simulink model "SecRwRtStBkReclnTrgtPosSelc"  (R2018b)
settings: Solver=FixedStepDiscrete  StartTime=0.0  StopTime=10.0  FixedStep=0.01  RelTol=1e-3
undefined symbols (not defined in the file or in its folder): KeSMSw4SAcsMd23SecRwRtStBkReclnUpwdDnwdPos_Val, KeSMSw4SAcsMd23SecRwRtStBkReclnUpwdDnwdPosMax_Val, KeSMSw4SAcsMd23SecRwRtStBkReclnUpwdDnwdPosMin_Val, KeSMSw4SAcsMd24SecRwRtStBkReclnUpwdDnwdPos1_Val, KeSMSw4SAcsMd24SecRwRtStBkReclnUpwdDnwdPos2_Val, KeSMSw4SAcsMd24SecRwRtStBkReclnUpwdDnwdPosMax1_Val, KeSMSw4SAcsMd24SecRwRtStBkReclnUpwdDnwdPosMax2_Val, KeSMSw4SAcsMd24SecRwRtStBkReclnUpwdDnwdPosMin1_Val, KeSMSw4SAcsMd24SecRwRtStBkReclnUpwdDnwdPosMin2_Val, KeSMSw4SAcsMd25SecRwRtStBkReclnUpwdDnwdPos_Val, KeSMSw4SAcsMd25SecRwRtStBkReclnUpwdDnwdPosMax_Val, KeSMSw4SAcsMd25SecRwRtStBkReclnUpwdDnwdPosMin_Val, KeSMSw4SAcsMd26SecRwRtStBkReclnUpwdDnwdPos_Val, KeSMSw4SAcsMd26SecRwRtStBkReclnUpwdDnwdPosMax_Val, KeSMSw4SAcsMd26SecRwRtStBkReclnUpwdDnwdPosMin_Val, KeSMSw4sLyingMDSecRwRtStBkReclnUpwdDnwdPos_Val, KeSMSw4sLyingMDSecRwRtStBkReclnUpwdDnwdPosMax_Val, KeSMSw4sLyingMDSecRwRtStBkReclnUpwdDnwdPosMin_Val, KeSMSw4sRecoveryMDSecRwRtStBkReclnUpwdDnwdPos_Val, KeSMSw4sRecoveryMDSecRwRtStBkReclnUpwdDnwdPosMax_Val, KeSMSw4sRecoveryMDSecRwRtStBkReclnUpwdDnwdPosMin_Val, KeSMSw4sVIPMDSecRwRtStBkReclnUpwdDnwdPos_Val, KeSMSw4sVIPMDSecRwRtStBkReclnUpwdDnwdPosMax_Val, KeSMSw4sVIPMDSecRwRtStBkReclnUpwdDnwdPosMin_Val, KeSMSw6sAcsEntrySecRwRtStBkReclnUpwdDnwd1Pos_Val, KeSMSw6sAcsEntrySecRwRtStBkReclnUpwdDnwdPos1Max_Val, KeSMSw6sAcsEntrySecRwRtStBkReclnUpwdDnwdPos1Min_Val, KeSMSw6sAcsEntrySecRwRtStBkReclnUpwdDnwdPos_Val, KeSMSw6sAcsEntrySecRwRtStBkReclnUpwdDnwdPosMax_Val, KeSMSw6sAcsEntrySecRwRtStBkReclnUpwdDnwdPosMin_Val, KeSMSw6sAcsExtSecRwRtStBkReclnUpwdDnwdPos_Val, KeSMSw6sAcsExtSecRwRtStBkReclnUpwdDnwdPosMax_Val, KeSMSw6sAcsExtSecRwRtStBkReclnUpwdDnwdPosMin_Val, KeSMSw6sRecoveryMdSecRwRtStBkReclnUpwdDnwdPos_Val, KeSMSw6sRecoveryMdSecRwRtStBkReclnUpwdDnwdPosMax_Val, KeSMSw6sRecoveryMdSecRwRtStBkReclnUpwdDnwdPosMin_Val, KeSMSw6sVIPSecRwRtStBkReclnUpwdDnwdPos_Val, KeSMSw6sVIPSecRwRtStBkReclnUpwdDnwdPosMax_Val, KeSMSw6sVIPSecRwRtStBkReclnUpwdDnwdPosMin_Val, KeSMSwAcsEntrySecRwRtStBkReclnUpwdDnwdPos1_Val, KeSMSwAcsEntrySecRwRtStBkReclnUpwdDnwdPos1Max_Val, KeSMSwAcsEntrySecRwRtStBkReclnUpwdDnwdPos1Min_Val, KeSMSwAcsEntrySecRwRtStBkReclnUpwdDnwdPos_Val, KeSMSwAcsEntrySecRwRtStBkReclnUpwdDnwdPosMax_Val, KeSMSwAcsEntrySecRwRtStBkReclnUpwdDnwdPosMin_Val, KeSMSwAcsExtSecRwRtStBkReclnUpwdDnwdPos_Val, KeSMSwAcsExtSecRwRtStBkReclnUpwdDnwdPosMax_Val, KeSMSwAcsExtSecRwRtStBkReclnUpwdDnwdPosMin_Val, KeSMSwAcsMd32SecRwRtStBkReclnUpwdDnwdPos1_Val, KeSMSwAcsMd32SecRwRtStBkReclnUpwdDnwdPos1Max_Val, KeSMSwAcsMd32SecRwRtStBkReclnUpwdDnwdPos1Min_Val, KeSMSwAcsMd32SecRwRtStBkReclnUpwdDnwdPos_Val, KeSMSwAcsMd32SecRwRtStBkReclnUpwdDnwdPosMax_Val, KeSMSwAcsMd32SecRwRtStBkReclnUpwdDnwdPosMin_Val, KeSMSwAcsMd53SecRwRtStBkReclnUpwdDnwdPos1_Val, KeSMSwAcsMd53SecRwRtStBkReclnUpwdDnwdPos1Max_Val, KeSMSwAcsMd53SecRwRtStBkReclnUpwdDnwdPos1Min_Val, KeSMSwAcsMd53SecRwRtStBkReclnUpwdDnwdPos_Val, KeSMSwAcsMd53SecRwRtStBkReclnUpwdDnwdPosMax_Val, KeSMSwAcsMd53SecRwRtStBkReclnUpwdDnwdPosMin_Val ... (+12)
libraries: TrgtPosSelcLib x15, simulink x2
(part 2 of 2)

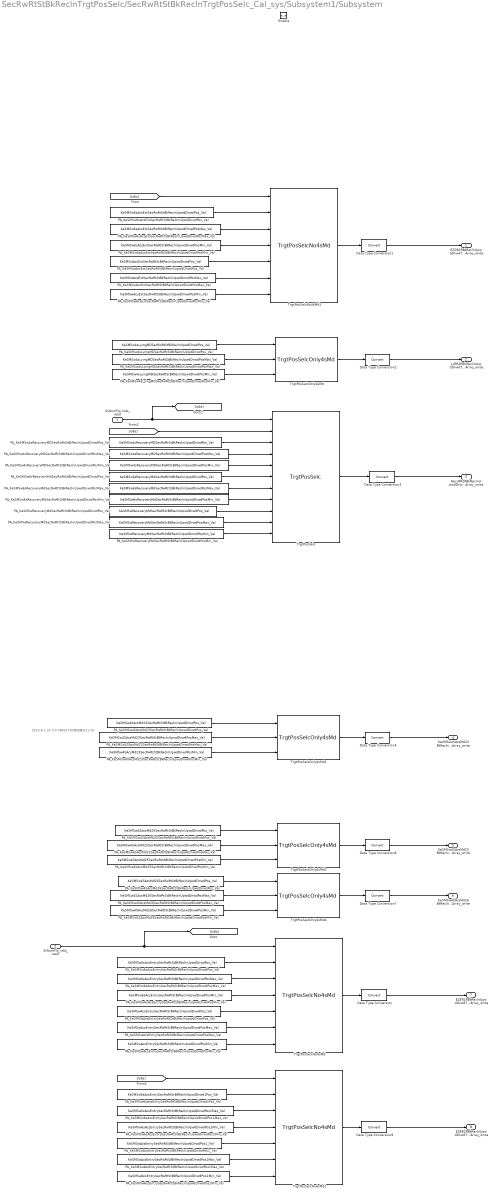
== system SecRwRtStBkReclnTrgtPosSelc/SecRwRtStBkReclnTrgtPosSelc_Cal_sys/Subsystem1/Subsystem ==
  note: 2023.8.1 V2.0.0 CR401790 增加模式21-26
  StNumFlg_Is4s_read : Inport
  StNumFlg_Is6s_read : Inport  Port=2
  Enable : EnablePort
  Data Type Conversion{,1..3,5..8} (8 alike) : DataTypeConversion
  PA_KeSMSw4SAcsMd23SecRwRtStBkReclnUpwdDnwdPosMax_Val : Constant  Value=KeSMSw4SAcsMd23SecRwRtStBkReclnUpwdDnwdPosMax_Val
  PA_KeSMSw4SAcsMd23SecRwRtStBkReclnUpwdDnwdPosMin_Val : Constant  Value=KeSMSw4SAcsMd23SecRwRtStBkReclnUpwdDnwdPosMin_Val
  PA_KeSMSw4SAcsMd23SecRwRtStBkReclnUpwdDnwdPos_Val : Constant  Value=KeSMSw4SAcsMd23SecRwRtStBkReclnUpwdDnwdPos_Val
  PA_KeSMSw4SAcsMd25SecRwRtStBkReclnUpwdDnwdPosMax_Val : Constant  Value=KeSMSw4SAcsMd25SecRwRtStBkReclnUpwdDnwdPosMax_Val
  PA_KeSMSw4SAcsMd25SecRwRtStBkReclnUpwdDnwdPosMin_Val : Constant  Value=KeSMSw4SAcsMd25SecRwRtStBkReclnUpwdDnwdPosMin_Val
  PA_KeSMSw4SAcsMd25SecRwRtStBkReclnUpwdDnwdPos_Val : Constant  Value=KeSMSw4SAcsMd25SecRwRtStBkReclnUpwdDnwdPos_Val
  PA_KeSMSw4SAcsMd26SecRwRtStBkReclnUpwdDnwdPosMax_Val : Constant  Value=KeSMSw4SAcsMd26SecRwRtStBkReclnUpwdDnwdPosMax_Val
  PA_KeSMSw4SAcsMd26SecRwRtStBkReclnUpwdDnwdPosMin_Val : Constant  Value=KeSMSw4SAcsMd26SecRwRtStBkReclnUpwdDnwdPosMin_Val
  PA_KeSMSw4SAcsMd26SecRwRtStBkReclnUpwdDnwdPos_Val : Constant  Value=KeSMSw4SAcsMd26SecRwRtStBkReclnUpwdDnwdPos_Val
  PA_KeSMSw4sLyingMDSecRwRtStBkReclnUpwdDnwdPosMax_Val : Constant  Value=KeSMSw4sLyingMDSecRwRtStBkReclnUpwdDnwdPosMax_Val
  PA_KeSMSw4sLyingMDSecRwRtStBkReclnUpwdDnwdPosMin_Val : Constant  Value=KeSMSw4sLyingMDSecRwRtStBkReclnUpwdDnwdPosMin_Val
  PA_KeSMSw4sLyingMDSecRwRtStBkReclnUpwdDnwdPos_Val : Constant  Value=KeSMSw4sLyingMDSecRwRtStBkReclnUpwdDnwdPos_Val
  PA_KeSMSw4sRecoveryMDSecRwRtStBkReclnUpwdDnwdPosMax_Val : Constant  Value=KeSMSw4sRecoveryMDSecRwRtStBkReclnUpwdDnwdPosMax_Val
  PA_KeSMSw4sRecoveryMDSecRwRtStBkReclnUpwdDnwdPosMin_Val : Constant  Value=KeSMSw4sRecoveryMDSecRwRtStBkReclnUpwdDnwdPosMin_Val
  PA_KeSMSw4sRecoveryMDSecRwRtStBkReclnUpwdDnwdPos_Val : Constant  Value=KeSMSw4sRecoveryMDSecRwRtStBkReclnUpwdDnwdPos_Val
  PA_KeSMSw6sAcsEntrySecRwRtStBkReclnUpwdDnwd1Pos_Val : Constant  Value=KeSMSw6sAcsEntrySecRwRtStBkReclnUpwdDnwd1Pos_Val
  PA_KeSMSw6sAcsEntrySecRwRtStBkReclnUpwdDnwdPos1Max_Val : Constant  Value=KeSMSw6sAcsEntrySecRwRtStBkReclnUpwdDnwdPos1Max_Val
  PA_KeSMSw6sAcsEntrySecRwRtStBkReclnUpwdDnwdPos1Min_Val : Constant  Value=KeSMSw6sAcsEntrySecRwRtStBkReclnUpwdDnwdPos1Min_Val
  PA_KeSMSw6sAcsEntrySecRwRtStBkReclnUpwdDnwdPosMax_Val : Constant  Value=KeSMSw6sAcsEntrySecRwRtStBkReclnUpwdDnwdPosMax_Val
  PA_KeSMSw6sAcsEntrySecRwRtStBkReclnUpwdDnwdPosMin_Val : Constant  Value=KeSMSw6sAcsEntrySecRwRtStBkReclnUpwdDnwdPosMin_Val
  PA_KeSMSw6sAcsEntrySecRwRtStBkReclnUpwdDnwdPos_Val : Constant  Value=KeSMSw6sAcsEntrySecRwRtStBkReclnUpwdDnwdPos_Val
  PA_KeSMSw6sAcsExtSecRwRtStBkReclnUpwdDnwdPosMax_Val : Constant  Value=KeSMSw6sAcsExtSecRwRtStBkReclnUpwdDnwdPosMax_Val
  PA_KeSMSw6sAcsExtSecRwRtStBkReclnUpwdDnwdPosMin_Val : Constant  Value=KeSMSw6sAcsExtSecRwRtStBkReclnUpwdDnwdPosMin_Val
  PA_KeSMSw6sAcsExtSecRwRtStBkReclnUpwdDnwdPos_Val : Constant  Value=KeSMSw6sAcsExtSecRwRtStBkReclnUpwdDnwdPos_Val
  PA_KeSMSw6sRecoveryMdSecRwRtStBkReclnUpwdDnwdPosMax_Val : Constant  Value=KeSMSw6sRecoveryMdSecRwRtStBkReclnUpwdDnwdPosMax_Val
  PA_KeSMSw6sRecoveryMdSecRwRtStBkReclnUpwdDnwdPosMin_Val : Constant  Value=KeSMSw6sRecoveryMdSecRwRtStBkReclnUpwdDnwdPosMin_Val
  PA_KeSMSw6sRecoveryMdSecRwRtStBkReclnUpwdDnwdPos_Val : Constant  Value=KeSMSw6sRecoveryMdSecRwRtStBkReclnUpwdDnwdPos_Val
  PA_KeSMSwAcsEntrySecRwRtStBkReclnUpwdDnwdPos1Max_Val : Constant  Value=KeSMSwAcsEntrySecRwRtStBkReclnUpwdDnwdPos1Max_Val
  PA_KeSMSwAcsEntrySecRwRtStBkReclnUpwdDnwdPos1Min_Val : Constant  Value=KeSMSwAcsEntrySecRwRtStBkReclnUpwdDnwdPos1Min_Val
  PA_KeSMSwAcsEntrySecRwRtStBkReclnUpwdDnwdPos1_Val : Constant  Value=KeSMSwAcsEntrySecRwRtStBkReclnUpwdDnwdPos1_Val
  PA_KeSMSwAcsEntrySecRwRtStBkReclnUpwdDnwdPosMax_Val : Constant  Value=KeSMSwAcsEntrySecRwRtStBkReclnUpwdDnwdPosMax_Val
  PA_KeSMSwAcsEntrySecRwRtStBkReclnUpwdDnwdPosMin_Val : Constant  Value=KeSMSwAcsEntrySecRwRtStBkReclnUpwdDnwdPosMin_Val
  PA_KeSMSwAcsEntrySecRwRtStBkReclnUpwdDnwdPos_Val : Constant  Value=KeSMSwAcsEntrySecRwRtStBkReclnUpwdDnwdPos_Val
  PA_KeSMSwAcsExtSecRwRtStBkReclnUpwdDnwdPosMax_Val : Constant  Value=KeSMSwAcsExtSecRwRtStBkReclnUpwdDnwdPosMax_Val
  PA_KeSMSwAcsExtSecRwRtStBkReclnUpwdDnwdPosMin_Val : Constant  Value=KeSMSwAcsExtSecRwRtStBkReclnUpwdDnwdPosMin_Val
  PA_KeSMSwAcsExtSecRwRtStBkReclnUpwdDnwdPos_Val : Constant  Value=KeSMSwAcsExtSecRwRtStBkReclnUpwdDnwdPos_Val
  PA_KeSMSwRecoveryMdSecRwRtStBkReclnUpwdDnwdPosMax_Val : Constant  Value=KeSMSwRecoveryMdSecRwRtStBkReclnUpwdDnwdPosMax_Val
  PA_KeSMSwRecoveryMdSecRwRtStBkReclnUpwdDnwdPosMin_Val : Constant  Value=KeSMSwRecoveryMdSecRwRtStBkReclnUpwdDnwdPosMin_Val
  PA_KeSMSwRecoveryMdSecRwRtStBkReclnUpwdDnwdPos_Val : Constant  Value=KeSMSwRecoveryMdSecRwRtStBkReclnUpwdDnwdPos_Val
  TrgtPosSelc : TrgtPosSelcLib/TrgtPosSelc  SystemSampleTime=-1
  TrgtPosSelcNo4sMd : TrgtPosSelcLib/TrgtPosSelcNo4sMd  SystemSampleTime=-1
  TrgtPosSelcNo4sMd1 : TrgtPosSelcLib/TrgtPosSelcNo4sMd  SystemSampleTime=-1
  TrgtPosSelcNo4sMd2 : TrgtPosSelcLib/TrgtPosSelcNo4sMd  SystemSampleTime=-1
  TrgtPosSelcOnly4sMd{,1,3..4} (4 alike) : TrgtPosSelcLib/TrgtPosSelcOnly4sMd  SystemSampleTime=-1
  EZQR2RBkReclnUpwdDnwdTrgtPosCalib_TrgtPosArray_write : Outport
  LyRR2RBkReclnUpwdDnwdTrgtPosCalib_TrgtPosArray_write : Outport  Port=2
  RecvRR2RBkReclnUpwdDnwdTrgtPosCalib_TrgtPosArray_write : Outport  Port=3
  KeSMSw4SAcsMd23BkReclnUpwdDnwdTrgtPosCalib_TrgtPosArray_write : Outport  Port=4
  KeSMSw4SAcsMd25BkReclnUpwdDnwdTrgtPosCalib_TrgtPosArray_write : Outport  Port=5
  KeSMSw4SAcsMd26BkReclnUpwdDnwdTrgtPosCalib_TrgtPosArray_write : Outport  Port=6
  EZER2RBkReclnUpwdDnwdTrgtPosCalib_TrgtPosArray_write : Outport  Port=7
  EZER2RBkReclnUpwdDnwdTrgtPosCalib1_TrgtPosArray_write : Outport  Port=8
  wires:
  StNumFlg_Is6s_read/1 -> [Is6s], TrgtPosSelcNo4sMd/1
  PA_KeSMSw6sAcsExtSecRwRtStBkReclnUpwdDnwdPosMin_Val/1 -> TrgtPosSelcNo4sMd1/4
  StNumFlg_Is4s_read/1 -> [Is4s], TrgtPosSelc/1
  PA_KeSMSw6sAcsEntrySecRwRtStBkReclnUpwdDnwdPosMin_Val/1 -> TrgtPosSelcNo4sMd/4
  PA_KeSMSw6sAcsExtSecRwRtStBkReclnUpwdDnwdPosMax_Val/1 -> TrgtPosSelcNo4sMd1/3
  PA_KeSMSw4sLyingMDSecRwRtStBkReclnUpwdDnwdPos_Val/1 -> TrgtPosSelcOnly4sMd/1
  PA_KeSMSw6sAcsExtSecRwRtStBkReclnUpwdDnwdPos_Val/1 -> TrgtPosSelcNo4sMd1/2
  PA_KeSMSw6sAcsEntrySecRwRtStBkReclnUpwdDnwdPos_Val/1 -> TrgtPosSelcNo4sMd/2
  TrgtPosSelcNo4sMd1/1 -> Data Type Conversion1/1
  PA_KeSMSw6sAcsEntrySecRwRtStBkReclnUpwdDnwdPosMax_Val/1 -> TrgtPosSelcNo4sMd/3
  TrgtPosSelcNo4sMd/1 -> Data Type Conversion/1
  TrgtPosSelc/1 -> Data Type Conversion3/1
  TrgtPosSelcOnly4sMd/1 -> Data Type Conversion2/1
  [Is6s] -> TrgtPosSelcNo4sMd1/1
  PA_KeSMSw4sLyingMDSecRwRtStBkReclnUpwdDnwdPosMax_Val/1 -> TrgtPosSelcOnly4sMd/2
  PA_KeSMSw4sLyingMDSecRwRtStBkReclnUpwdDnwdPosMin_Val/1 -> TrgtPosSelcOnly4sMd/3
  [Is6s] -> TrgtPosSelc/2
  PA_KeSMSw6sRecoveryMdSecRwRtStBkReclnUpwdDnwdPos_Val/1 -> TrgtPosSelc/6
  PA_KeSMSw6sRecoveryMdSecRwRtStBkReclnUpwdDnwdPosMax_Val/1 -> TrgtPosSelc/7
  PA_KeSMSw6sRecoveryMdSecRwRtStBkReclnUpwdDnwdPosMin_Val/1 -> TrgtPosSelc/8
  PA_KeSMSwAcsEntrySecRwRtStBkReclnUpwdDnwdPosMin_Val/1 -> TrgtPosSelcNo4sMd/7
  PA_KeSMSwAcsEntrySecRwRtStBkReclnUpwdDnwdPosMax_Val/1 -> TrgtPosSelcNo4sMd/6
  PA_KeSMSwAcsEntrySecRwRtStBkReclnUpwdDnwdPos_Val/1 -> TrgtPosSelcNo4sMd/5
  PA_KeSMSwAcsExtSecRwRtStBkReclnUpwdDnwdPosMin_Val/1 -> TrgtPosSelcNo4sMd1/7
  PA_KeSMSwAcsExtSecRwRtStBkReclnUpwdDnwdPosMax_Val/1 -> TrgtPosSelcNo4sMd1/6
  PA_KeSMSwAcsExtSecRwRtStBkReclnUpwdDnwdPos_Val/1 -> TrgtPosSelcNo4sMd1/5
  PA_KeSMSw4sRecoveryMDSecRwRtStBkReclnUpwdDnwdPos_Val/1 -> TrgtPosSelc/3
  PA_KeSMSw4sRecoveryMDSecRwRtStBkReclnUpwdDnwdPosMax_Val/1 -> TrgtPosSelc/4
  PA_KeSMSw4sRecoveryMDSecRwRtStBkReclnUpwdDnwdPosMin_Val/1 -> TrgtPosSelc/5
  PA_KeSMSwRecoveryMdSecRwRtStBkReclnUpwdDnwdPosMax_Val/1 -> TrgtPosSelc/10
  PA_KeSMSwRecoveryMdSecRwRtStBkReclnUpwdDnwdPosMin_Val/1 -> TrgtPosSelc/11
  PA_KeSMSwRecoveryMdSecRwRtStBkReclnUpwdDnwdPos_Val/1 -> TrgtPosSelc/9
  TrgtPosSelcOnly4sMd1/1 -> Data Type Conversion5/1
  TrgtPosSelcOnly4sMd3/1 -> Data Type Conversion6/1
  TrgtPosSelcOnly4sMd4/1 -> Data Type Conversion7/1
  PA_KeSMSw4SAcsMd23SecRwRtStBkReclnUpwdDnwdPos_Val/1 -> TrgtPosSelcOnly4sMd1/1
  PA_KeSMSw4SAcsMd23SecRwRtStBkReclnUpwdDnwdPosMax_Val/1 -> TrgtPosSelcOnly4sMd1/2
  PA_KeSMSw4SAcsMd23SecRwRtStBkReclnUpwdDnwdPosMin_Val/1 -> TrgtPosSelcOnly4sMd1/3
  PA_KeSMSw4SAcsMd25SecRwRtStBkReclnUpwdDnwdPos_Val/1 -> TrgtPosSelcOnly4sMd3/1
  PA_KeSMSw4SAcsMd25SecRwRtStBkReclnUpwdDnwdPosMax_Val/1 -> TrgtPosSelcOnly4sMd3/2
  PA_KeSMSw4SAcsMd25SecRwRtStBkReclnUpwdDnwdPosMin_Val/1 -> TrgtPosSelcOnly4sMd3/3
  PA_KeSMSw4SAcsMd26SecRwRtStBkReclnUpwdDnwdPos_Val/1 -> TrgtPosSelcOnly4sMd4/1
  PA_KeSMSw4SAcsMd26SecRwRtStBkReclnUpwdDnwdPosMax_Val/1 -> TrgtPosSelcOnly4sMd4/2
  PA_KeSMSw4SAcsMd26SecRwRtStBkReclnUpwdDnwdPosMin_Val/1 -> TrgtPosSelcOnly4sMd4/3
  Data Type Conversion/1 -> EZER2RBkReclnUpwdDnwdTrgtPosCalib_TrgtPosArray_write/1
  Data Type Conversion1/1 -> EZQR2RBkReclnUpwdDnwdTrgtPosCalib_TrgtPosArray_write/1
  Data Type Conversion2/1 -> LyRR2RBkReclnUpwdDnwdTrgtPosCalib_TrgtPosArray_write/1
  Data Type Conversion3/1 -> RecvRR2RBkReclnUpwdDnwdTrgtPosCalib_TrgtPosArray_write/1
  Data Type Conversion5/1 -> KeSMSw4SAcsMd23BkReclnUpwdDnwdTrgtPosCalib_TrgtPosArray_write/1
  Data Type Conversion6/1 -> KeSMSw4SAcsMd25BkReclnUpwdDnwdTrgtPosCalib_TrgtPosArray_write/1
  Data Type Conversion7/1 -> KeSMSw4SAcsMd26BkReclnUpwdDnwdTrgtPosCalib_TrgtPosArray_write/1
  TrgtPosSelcNo4sMd2/1 -> Data Type Conversion8/1
  Data Type Conversion8/1 -> EZER2RBkReclnUpwdDnwdTrgtPosCalib1_TrgtPosArray_write/1
  [Is6s] -> TrgtPosSelcNo4sMd2/1
  PA_KeSMSwAcsEntrySecRwRtStBkReclnUpwdDnwdPos1Min_Val/1 -> TrgtPosSelcNo4sMd2/7
  PA_KeSMSwAcsEntrySecRwRtStBkReclnUpwdDnwdPos1Max_Val/1 -> TrgtPosSelcNo4sMd2/6
  PA_KeSMSw6sAcsEntrySecRwRtStBkReclnUpwdDnwdPos1Min_Val/1 -> TrgtPosSelcNo4sMd2/4
  PA_KeSMSw6sAcsEntrySecRwRtStBkReclnUpwdDnwdPos1Max_Val/1 -> TrgtPosSelcNo4sMd2/3
  PA_KeSMSwAcsEntrySecRwRtStBkReclnUpwdDnwdPos1_Val/1 -> TrgtPosSelcNo4sMd2/5
  PA_KeSMSw6sAcsEntrySecRwRtStBkReclnUpwdDnwd1Pos_Val/1 -> TrgtPosSelcNo4sMd2/2

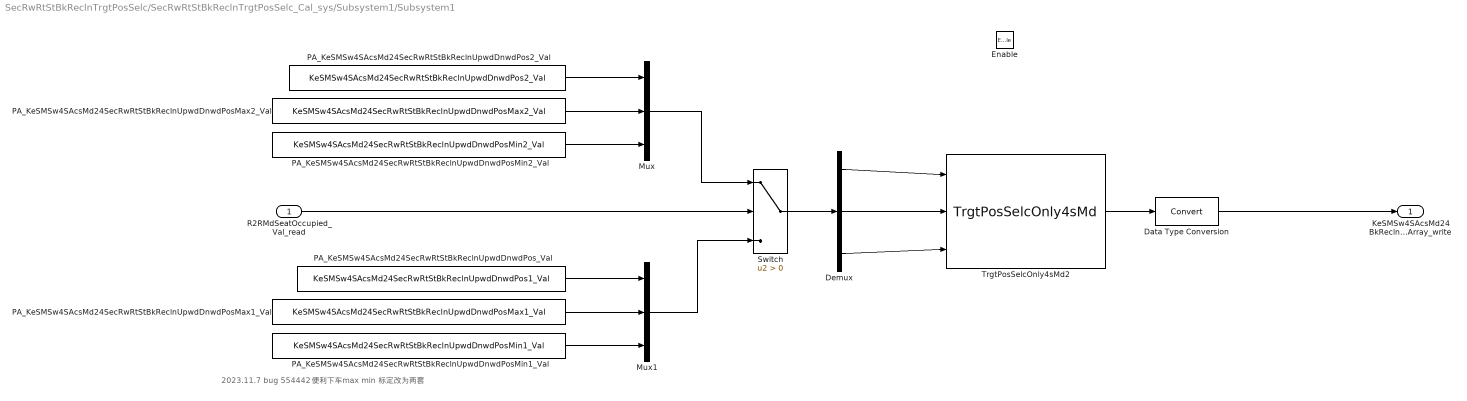
== system SecRwRtStBkReclnTrgtPosSelc/SecRwRtStBkReclnTrgtPosSelc_Cal_sys/Subsystem1/Subsystem1 ==
  note: 2023.11.7 bug 554442 便利下车max min 标定改为两套
  R2RMdSeatOccupied_Val_read : Inport
  Enable : EnablePort
  Data Type Conversion : DataTypeConversion
  Demux : Demux  Outputs=3
  Mux : Mux  Inputs=3
  Mux1 : Mux  Inputs=3
  PA_KeSMSw4SAcsMd24SecRwRtStBkReclnUpwdDnwdPos2_Val : Constant  Value=KeSMSw4SAcsMd24SecRwRtStBkReclnUpwdDnwdPos2_Val
  PA_KeSMSw4SAcsMd24SecRwRtStBkReclnUpwdDnwdPosMax1_Val : Constant  Value=KeSMSw4SAcsMd24SecRwRtStBkReclnUpwdDnwdPosMax1_Val
  PA_KeSMSw4SAcsMd24SecRwRtStBkReclnUpwdDnwdPosMax2_Val : Constant  Value=KeSMSw4SAcsMd24SecRwRtStBkReclnUpwdDnwdPosMax2_Val
  PA_KeSMSw4SAcsMd24SecRwRtStBkReclnUpwdDnwdPosMin1_Val : Constant  Value=KeSMSw4SAcsMd24SecRwRtStBkReclnUpwdDnwdPosMin1_Val
  PA_KeSMSw4SAcsMd24SecRwRtStBkReclnUpwdDnwdPosMin2_Val : Constant  Value=KeSMSw4SAcsMd24SecRwRtStBkReclnUpwdDnwdPosMin2_Val
  PA_KeSMSw4SAcsMd24SecRwRtStBkReclnUpwdDnwdPos_Val : Constant  Value=KeSMSw4SAcsMd24SecRwRtStBkReclnUpwdDnwdPos1_Val
  Switch : Switch  Criteria=u2 > Threshold
  TrgtPosSelcOnly4sMd2 : TrgtPosSelcLib/TrgtPosSelcOnly4sMd  SystemSampleTime=-1
  KeSMSw4SAcsMd24BkReclnUpwdDnwdTrgtPosCalib_TrgtPosArray_write : Outport
  wires:
  TrgtPosSelcOnly4sMd2/1 -> Data Type Conversion/1
  R2RMdSeatOccupied_Val_read/1 -> Switch/2
  Data Type Conversion/1 -> KeSMSw4SAcsMd24BkReclnUpwdDnwdTrgtPosCalib_TrgtPosArray_write/1
  PA_KeSMSw4SAcsMd24SecRwRtStBkReclnUpwdDnwdPosMax1_Val/1 -> Mux1/2
  Switch/1 -> Demux/1
  Demux/1 -> TrgtPosSelcOnly4sMd2/1
  Demux/2 -> TrgtPosSelcOnly4sMd2/2
  Demux/3 -> TrgtPosSelcOnly4sMd2/3
  Mux/1 -> Switch/1
  PA_KeSMSw4SAcsMd24SecRwRtStBkReclnUpwdDnwdPos2_Val/1 -> Mux/1
  PA_KeSMSw4SAcsMd24SecRwRtStBkReclnUpwdDnwdPosMax2_Val/1 -> Mux/2
  PA_KeSMSw4SAcsMd24SecRwRtStBkReclnUpwdDnwdPosMin2_Val/1 -> Mux/3
  Mux1/1 -> Switch/3
  PA_KeSMSw4SAcsMd24SecRwRtStBkReclnUpwdDnwdPos_Val/1 -> Mux1/1
  PA_KeSMSw4SAcsMd24SecRwRtStBkReclnUpwdDnwdPosMin1_Val/1 -> Mux1/3

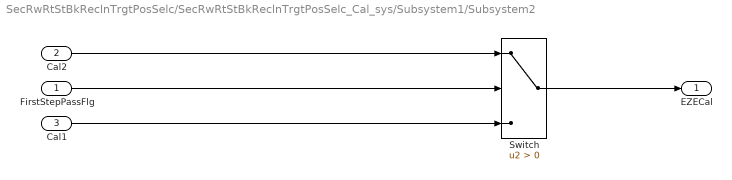
== system SecRwRtStBkReclnTrgtPosSelc/SecRwRtStBkReclnTrgtPosSelc_Cal_sys/Subsystem1/Subsystem2 ==
  FirstStepPassFlg : Inport
  Cal2 : Inport  Port=2
  Cal1 : Inport  Port=3
  Switch : Switch  Criteria=u2 > Threshold
  EZECal : Outport
  wires:
  Switch/1 -> EZECal/1
  FirstStepPassFlg/1 -> Switch/2
  Cal2/1 -> Switch/1
  Cal1/1 -> Switch/3
